simulink model "irep_force_control_m15"  (R2015a)
settings: Solver=ode3  StartTime=0.0  StopTime=inf  FixedStep=dt  RelTol=1e-3
InitFcn:
  | IREP_DEPENDENCY
  | init_omni
  | init_filters
  | init_invivo
  | init_telemanipulation
  | init_parker_xyz
  | init_magnetic_tracker
  | init_loadcell
  | init_scopes
  | init_homing
  | init_force_control
  | init_xpc_invivo_simu
undefined symbols (not defined in the file): ang_vel_scale, B_simu, beta, camera_home_voltage, counter_offset, dt, dt_trakstar, E_Y, encoder_counts, epsilon_robust_inverse, FS_LUT_TAU, FS_LUT_WE, gear_ratio, HomingFineEps, HomingRoughEps, HomingRoughVelocity, I1_primary, I1_secondary, I2_primary, I2_secondary, irep_parameters_left, irep_parameters_right, joystick_filter_coeffs, K_d, K_i, K_naive_inv, K_p, k_right, L1l, L1r, L2l, L2r, L_zeus, left_arm_home_voltage, left_x0_parallelogram, LeftArmHomingDirectionVector, LeftArmHomingIntGain, lin_vel_scale, LOADCELL_BIAS, LOADCELL_GAIN, max_conf_space_speed, N_joystick, N_pots, N_trakstar, OmegaMax, OmegaMin, orientation_epsilon, position_epsilon, pots_filter_coeffs, q_eps_backlash, quadrature_mode, r, right_arm_home_voltage, RightArmHomingDirectionVector, RightArmHomingIntGain, screw_pitch, statics_param, tau_compression_bias, tau_compression_gains, tau_neutral_deadband ... (+16)
libraries: slrtlib x39, simulink x23, xpcobsoletelib x23, xpcconteclib x23, xpcrtudplib x12, xpcmeasurementcomputinglib x6, dspswit3 x2, dspsigops x1
(part 3 of 7)

== system irep_force_control_m15/In-Vivo System/CONTEC CARDS/Level 3 ==
  note: Contec
      | CNT32-8M (PCI)
      | Inc. Encoder
      | Slot: [2, 11]
      | channel [1,4,5,6,7]
  Mux : Mux  Inputs=5
  camera: open joint : xpcconteclib/Incremental Encoder/CNT32-8M(PCI)   Channel=5  OperationMode=2-phase Input Synchronous Clear Multiply by 4  DigitalFilter=No filtering  PulseInput=TTL level input  Direction=Up in the clockwise direction/Down in the counterclockwise direction  InitialValue=counter_offset_init  LoadInitialValue=on  SampleTime=dt  PciSlot=[2,11]  StartMethod=Model Start  StopMethod=Model Terminate  ZeroClearRising=off  ZeroClearFalling=off  ZeroClearMatch0=off  ZeroClearMatch1=off  PresetRising=off  PresetFalling=off  PresetMatch0=off  PresetMatch1=off  PresetValue=0  Match0Value=0  Match1Value=0  OutputSignalMatch0=off  OutputSignalMatch1=off  OutputSignalAbnormal=off  OutputSignalDigitalFilter=off  OutputSignalAlarm=off  OneShotDuration=10 microseconds  IndexEnable=Disable  IndexLogic=Positive (Active High)  EnableDigitalInput=off  EnableDigitalOutput=off  DigitalOutputInitialValue=None  DigitalOutputFinalValue=None
  camera: open joint1 : xpcconteclib/Incremental Encoder/CNT32-8M(PCI)   Channel=6  OperationMode=2-phase Input Synchronous Clear Multiply by 4  DigitalFilter=No filtering  PulseInput=TTL level input  Direction=Up in the clockwise direction/Down in the counterclockwise direction  InitialValue=counter_offset_init  LoadInitialValue=on  SampleTime=dt  PciSlot=[2,11]  StartMethod=Model Start  StopMethod=Model Terminate  ZeroClearRising=off  ZeroClearFalling=off  ZeroClearMatch0=off  ZeroClearMatch1=off  PresetRising=off  PresetFalling=off  PresetMatch0=off  PresetMatch1=off  PresetValue=0  Match0Value=0  Match1Value=0  OutputSignalMatch0=off  OutputSignalMatch1=off  OutputSignalAbnormal=off  OutputSignalDigitalFilter=off  OutputSignalAlarm=off  OneShotDuration=10 microseconds  IndexEnable=Disable  IndexLogic=Positive (Active High)  EnableDigitalInput=off  EnableDigitalOutput=off  DigitalOutputInitialValue=None  DigitalOutputFinalValue=None
  camera: open joint2 : xpcconteclib/Incremental Encoder/CNT32-8M(PCI)   Channel=7  OperationMode=2-phase Input Synchronous Clear Multiply by 4  DigitalFilter=No filtering  PulseInput=TTL level input  Direction=Up in the clockwise direction/Down in the counterclockwise direction  InitialValue=counter_offset_init  LoadInitialValue=on  SampleTime=dt  PciSlot=[2,11]  StartMethod=Model Start  StopMethod=Model Terminate  ZeroClearRising=off  ZeroClearFalling=off  ZeroClearMatch0=off  ZeroClearMatch1=off  PresetRising=off  PresetFalling=off  PresetMatch0=off  PresetMatch1=off  PresetValue=0  Match0Value=0  Match1Value=0  OutputSignalMatch0=off  OutputSignalMatch1=off  OutputSignalAbnormal=off  OutputSignalDigitalFilter=off  OutputSignalAlarm=off  OneShotDuration=10 microseconds  IndexEnable=Disable  IndexLogic=Positive (Active High)  EnableDigitalInput=off  EnableDigitalOutput=off  DigitalOutputInitialValue=None  DigitalOutputFinalValue=None
  left arm: insertion : xpcconteclib/Incremental Encoder/CNT32-8M(PCI)   Channel=4  OperationMode=2-phase Input Synchronous Clear Multiply by 4  DigitalFilter=No filtering  PulseInput=TTL level input  Direction=Up in the clockwise direction/Down in the counterclockwise direction  InitialValue=counter_offset_init  LoadInitialValue=on  SampleTime=dt  PciSlot=[2,11]  StartMethod=Model Start  StopMethod=Model Terminate  ZeroClearRising=off  ZeroClearFalling=off  ZeroClearMatch0=off  ZeroClearMatch1=off  PresetRising=off  PresetFalling=off  PresetMatch0=off  PresetMatch1=off  PresetValue=0  Match0Value=0  Match1Value=0  OutputSignalMatch0=off  OutputSignalMatch1=off  OutputSignalAbnormal=off  OutputSignalDigitalFilter=off  OutputSignalAlarm=off  OneShotDuration=10 microseconds  IndexEnable=Disable  IndexLogic=Positive (Active High)  EnableDigitalInput=off  EnableDigitalOutput=off  DigitalOutputInitialValue=None  DigitalOutputFinalValue=None
  right arm: insertion : xpcconteclib/Incremental Encoder/CNT32-8M(PCI)   Channel=1  OperationMode=2-phase Input Synchronous Clear Multiply by 4  DigitalFilter=No filtering  PulseInput=TTL level input  Direction=Up in the clockwise direction/Down in the counterclockwise direction  InitialValue=counter_offset_init  LoadInitialValue=on  SampleTime=dt  PciSlot=[2,11]  StartMethod=Model Start  StopMethod=Model Terminate  ZeroClearRising=off  ZeroClearFalling=off  ZeroClearMatch0=off  ZeroClearMatch1=off  PresetRising=on  PresetFalling=off  PresetMatch0=off  PresetMatch1=off  PresetValue=0  Match0Value=0  Match1Value=0  OutputSignalMatch0=off  OutputSignalMatch1=off  OutputSignalAbnormal=off  OutputSignalDigitalFilter=off  OutputSignalAlarm=off  OneShotDuration=10 microseconds  IndexEnable=Disable  IndexLogic=Positive (Active High)  EnableDigitalInput=off  EnableDigitalOutput=off  DigitalOutputInitialValue=None  DigitalOutputFinalValue=None
  Out1 : Outport
  wires:
  Mux/1 -> Out1/1
  right arm: insertion/1 -> Mux/1
  camera: open joint2/1 -> Mux/5
  camera: open joint/1 -> Mux/3
  left arm: insertion/1 -> Mux/2
  camera: open joint1/1 -> Mux/4

== system irep_force_control_m15/In-Vivo System/CONTEC CARDS/RZ ==
  note: Contec
      | CNT32-8M (PCI)
      | Inc. Encoder
      | Slot: [2, 14]
      | channel [1,2]
  CNT32-8M(PCI) Ch1 : xpcconteclib/Incremental Encoder/CNT32-8M(PCI)   Channel=1  OperationMode=2-phase Input Synchronous Clear Multiply by 4  DigitalFilter=No filtering  PulseInput=Differential line receiver input  Direction=Up in the clockwise direction/Down in the counterclockwise direction  InitialValue=counter_offset  LoadInitialValue=on  SampleTime=dt  PciSlot=[2 14]  StartMethod=Model Start  StopMethod=Model Terminate  ZeroClearRising=off  ZeroClearFalling=off  ZeroClearMatch0=off  ZeroClearMatch1=off  PresetRising=off  PresetFalling=off  PresetMatch0=off  PresetMatch1=off  PresetValue=0  Match0Value=0  Match1Value=0  OutputSignalMatch0=off  OutputSignalMatch1=off  OutputSignalAbnormal=off  OutputSignalDigitalFilter=off  OutputSignalAlarm=off  OneShotDuration=10 microseconds  IndexEnable=Disable  IndexLogic=Positive (Active High)  EnableDigitalInput=off  EnableDigitalOutput=off  DigitalOutputInitialValue=None  DigitalOutputFinalValue=None
  CNT32-8M(PCI) Ch2 : xpcconteclib/Incremental Encoder/CNT32-8M(PCI)   Channel=2  OperationMode=2-phase Input Synchronous Clear Multiply by 4  DigitalFilter=No filtering  PulseInput=Differential line receiver input  Direction=Up in the clockwise direction/Down in the counterclockwise direction  InitialValue=counter_offset  LoadInitialValue=on  SampleTime=dt  PciSlot=[2 14]  StartMethod=Model Start  StopMethod=Model Terminate  ZeroClearRising=off  ZeroClearFalling=off  ZeroClearMatch0=off  ZeroClearMatch1=off  PresetRising=off  PresetFalling=off  PresetMatch0=off  PresetMatch1=off  PresetValue=0  Match0Value=0  Match1Value=0  OutputSignalMatch0=off  OutputSignalMatch1=off  OutputSignalAbnormal=off  OutputSignalDigitalFilter=off  OutputSignalAlarm=off  OneShotDuration=10 microseconds  IndexEnable=Disable  IndexLogic=Positive (Active High)  EnableDigitalInput=off  EnableDigitalOutput=off  DigitalOutputInitialValue=None  DigitalOutputFinalValue=None
  Mux : Mux  Inputs=2
  Out1 : Outport
  wires:
  Mux/1 -> Out1/1
  CNT32-8M(PCI) Ch1/1 -> Mux/1
  CNT32-8M(PCI) Ch2/1 -> Mux/2

== system irep_force_control_m15/In-Vivo System/Count to mm/Bus Creator ==
  In1 : Inport
  Bus Creator : BusCreator  Inputs=23
  Demux : Demux  Outputs=23
  Out1 : Outport
  wires:
  Demux/1 -> Bus Creator/1  "Righ arm - Proximal segment - bending in Y"
  Demux/2 -> Bus Creator/2  "Right arm - Gripper Joint"
  Demux/3 -> Bus Creator/3  "Right arm - Proximal segment - bending in X"
  Demux/4 -> Bus Creator/4  "Right arm - distal segment - bending in X"
  Demux/5 -> Bus Creator/5  "Right arm - wrist"
  Demux/6 -> Bus Creator/6  "Right arm - distal segment - bending in Y"
  Demux/7 -> Bus Creator/7  "Right arm - parallelogram deployment joint"
  Demux/8 -> Bus Creator/8  "Right arm - parallelogram insert joint"
  Demux/9 -> Bus Creator/9  "Left arm - proximal segment - bending in Y"
  Demux/10 -> Bus Creator/10  "Left arm - gripper joint"
  Demux/11 -> Bus Creator/11  "Left arm - proximal segment - bending in X"
  Demux/12 -> Bus Creator/12  "Left arm - distal segment - bending in x"
  Demux/13 -> Bus Creator/13  "Left arm - wrist"
  Demux/14 -> Bus Creator/14  "Left arm - distal segment - bending in y"
  Demux/15 -> Bus Creator/15  "Left arm - parallelogram deployment joint"
  Demux/16 -> Bus Creator/16  "Left arm - parallelogram insert joint"
  Demux/17 -> Bus Creator/17  "Right arm - overall translational movement"
  Demux/18 -> Bus Creator/18  "Left arm - overall translational movement"
  Demux/19 -> Bus Creator/19  "Camera shell open"
  Demux/20 -> Bus Creator/20  "Camera Pan"
  Demux/21 -> Bus Creator/21  "Camera Tilt"
  Bus Creator/1 -> Out1/1
  In1/1 -> Demux/1
  Demux/22 -> Bus Creator/22  "Parker insertion stage"
  Demux/23 -> Bus Creator/23  "Parker rotary stage"

== system irep_force_control_m15/In-Vivo System/D//A/Bus Selector 1 ==
  In1 : Inport
  Bus Selector : BusSelector  OutputSignals=Right arm - Proximal Segment Y,Right arm - Gripper Joint,Right arm - Proximal Segment X,Right arm - Distal Segment X,Right arm - Wrist Joint,Right arm - Distal Segment Y,Right arm - Parallelogram Deploy,Right arm - Parallelogram Insert
  Gain{,1..3} (4 alike) : Gain  Gain=-1
  Mux : Mux  Inputs=8
  Out1 : Outport
  wires:
  Bus Selector/1 -> Mux/1  "<Right arm - Proximal Segment Y>"
  Bus Selector/2 -> Mux/2  "<Right arm - Gripper Joint>"
  Bus Selector/3 -> Gain/1  "<Right arm - Proximal Segment X>"
  Bus Selector/4 -> Gain1/1  "<Right arm - Distal Segment X>"
  Bus Selector/5 -> Mux/5  "<Right arm - Wrist Joint>"
  Bus Selector/6 -> Mux/6  "<Right arm - Distal Segment Y>"
  Bus Selector/7 -> Gain2/1  "<Right arm - Parallelogram Deploy>"
  Bus Selector/8 -> Gain3/1  "<Right arm - Parallelogram Insert>"
  In1/1 -> Bus Selector/1
  Mux/1 -> Out1/1
  Gain/1 -> Mux/3
  Gain1/1 -> Mux/4
  Gain2/1 -> Mux/7
  Gain3/1 -> Mux/8

== system irep_force_control_m15/In-Vivo System/D//A/Bus Selector 2 ==
  In1 : Inport
  Bus Selector : BusSelector  OutputSignals=Left arm - Proximal Segment Y,Left arm - Gripper Joint,Left arm - Proximal Segment X,Left arm - Distal Segment X,Left arm - Wrist Joint,Left arm - Distal Segment Y,Left arm - Parallelogram Deploy,Left arm - Parallelogram Insert
  Gain{1..4} (4 alike) : Gain  Gain=-1
  Mux : Mux  Inputs=8
  Out1 : Outport
  wires:
  Bus Selector/1 -> Gain1/1  "<Left arm - Proximal Segment Y>"
  Bus Selector/2 -> Mux/2  "<Left arm - Gripper Joint>"
  Bus Selector/4 -> Mux/4  "<Left arm - Distal Segment X>"
  Bus Selector/5 -> Mux/5  "<Left arm - Wrist Joint>"
  Bus Selector/6 -> Gain2/1  "<Left arm - Distal Segment Y>"
  Bus Selector/7 -> Gain3/1  "<Left arm - Parallelogram Deploy>"
  Bus Selector/8 -> Gain4/1  "<Left arm - Parallelogram Insert>"
  In1/1 -> Bus Selector/1
  Mux/1 -> Out1/1
  Bus Selector/3 -> Mux/3  "<Left arm - Proximal Segment X>"
  Gain1/1 -> Mux/1
  Gain2/1 -> Mux/6
  Gain3/1 -> Mux/7
  Gain4/1 -> Mux/8

== system irep_force_control_m15/In-Vivo System/D//A/Bus Selector 3 ==
  In1 : Inport
  Bus Selector : BusSelector  OutputSignals=Righ arm - Overall Translational Movement,Left arm - Overall Translational Movement,Camera shell open,Camera Pan,Camera Tilt
  Mux : Mux  Inputs=5
  Out1 : Outport
  wires:
  Mux/1 -> Out1/1
  In1/1 -> Bus Selector/1
  Bus Selector/1 -> Mux/1  "<Righ arm - Overall Translational Movement>"
  Bus Selector/2 -> Mux/2  "<Left arm - Overall Translational Movement>"
  Bus Selector/3 -> Mux/3  "<Camera shell open>"
  Bus Selector/4 -> Mux/4  "<Camera Pan>"
  Bus Selector/5 -> Mux/5  "<Camera Tilt>"

== system irep_force_control_m15/In-Vivo System/D//A/Level 1 ==
  note: Measurement Computing
      | PCI-DDA08/12 Analog Output
      | slot: [2, 7]
  In1 : Inport
  Demux1 : Demux  Outputs=8
  Level 1 : xpcmeasurementcomputinglib/D//A/PCI-DDA08 12   channel=[1,2,3,4,5,6,7,8]  range=[-10,-10,-10,-10,-10,-10,-10,-10]  reset=[1,1,1,1,1,1,1,1]  initValue=[0,0,0,0,0,0,0,0]  sampletime=dt  pci_dev=[2, 7]
  wires:
  In1/1 -> Demux1/1
  Demux1/1 -> Level 1/1
  Demux1/2 -> Level 1/2
  Demux1/3 -> Level 1/3
  Demux1/4 -> Level 1/4
  Demux1/5 -> Level 1/5
  Demux1/6 -> Level 1/6
  Demux1/7 -> Level 1/7
  Demux1/8 -> Level 1/8

== system irep_force_control_m15/In-Vivo System/D//A/Level 2 ==
  note: Measurement Computing
      | PCI-DDA08/12 Analog Output
      | Slot: [2, 10]
  In1 : Inport
  Demux2 : Demux  Outputs=8
  Level 2 : xpcmeasurementcomputinglib/D//A/PCI-DDA08 12   channel=[1,2,3,4,5,6,7,8]  range=[-10,-10,-10,-10,-10,-10,-10,-10]  reset=[1,1,1,1,1,1,1,1]  initValue=[0,0,0,0,0,0,0,0]  sampletime=dt  pci_dev=[2, 10]
  wires:
  In1/1 -> Demux2/1
  Demux2/1 -> Level 2/1
  Demux2/2 -> Level 2/2
  Demux2/3 -> Level 2/3
  Demux2/4 -> Level 2/4
  Demux2/5 -> Level 2/5
  Demux2/6 -> Level 2/6
  Demux2/7 -> Level 2/7
  Demux2/8 -> Level 2/8

== system irep_force_control_m15/In-Vivo System/D//A/Level 3 ==
  note: Measurement Computing
      | PCI-DDA08/12
      | Analog Ouput
      | Slot: [2, 13]
      | Channels [1,4,5,6,7]
  In1 : Inport
  Demux1 : Demux  Outputs=5
  Level 3 : xpcmeasurementcomputinglib/D//A/PCI-DDA08 12   channel=[1,2,3,4,5,6,7]  range=[-10,-10,-10,-10,-10,-10,-10]  reset=[1,1,1,1,1,1,1]  initValue=[0,0,0,0,0,0,0]  sampletime=dt  pci_dev=[2, 13]
  wires:
  In1/1 -> Demux1/1
  Demux1/1 -> Level 3/1
  Demux1/2 -> Level 3/4
  Demux1/3 -> Level 3/5
  Demux1/4 -> Level 3/6
  Demux1/5 -> Level 3/7

== system irep_force_control_m15/In-Vivo System/D//A/Parker Level ==
  note: Measurement Computing
      | PCI-DAS1602/12
      | Analog Output
      | Slot: [1, 14]
  In1 : Inport
  Bus Selector : BusSelector  OutputSignals=Parker insertion stage,Parker rotary stage
  Gain : Gain  Gain=-1
  Gain1 : Gain  Gain=-1
  "PCI-DAS1602 12 " : xpcobsoletelib/Measurement Computing obs/D//A/PCI-DAS1602 12   channel=[1 2]  range=[-10 -10]  reset=[1 1]  initValue=[0 0]  sampletime=dt  pci_dev=[1 14]
  wires:
  Bus Selector/2 -> Gain/1  "<Parker rotary stage>"
  Bus Selector/1 -> Gain1/1  "<Parker insertion stage>"
  In1/1 -> Bus Selector/1
  Gain1/1 -> "PCI-DAS1602 12 "/1
  Gain/1 -> "PCI-DAS1602 12 "/2

== system irep_force_control_m15/In-Vivo System/Loadcells/Loadcell Backbone Mapping ==
  note: This direction gain is needed for the following reason:
      | The load cell reading "+" meaning tension, i.e. pushing on the backbone.
      | Pushing in the statics formulation use "-".
      | So the loadcell sign is opposite to the statics formulation
  note: This mapping is documented on the wiki
      | http://arma.vuse.vanderbilt.edu/mediawiki/index.php/Force_Sensing,_In-Vivo_Project#Loadcell__Backbone_Mapping
  loadcell reading : Inport
  Demux : Demux  Outputs=8
  Mux : Mux  Inputs=8
  direction : Gain  Gain=-1
  tau backbones : Outport
  wires:
  loadcell reading/1 -> Demux/1
  Demux/1 -> [LC1]  "LC1"
  Demux/2 -> [LC2]  "LC2"
  Demux/3 -> [LC3]  "LC3"
  Demux/4 -> [LC4]  "LC4"
  Demux/5 -> [LC5]  "LC5"
  Demux/6 -> [LC6]  "LC6"
  Demux/7 -> [LC7]  "LC7"
  Demux/8 -> [LC8]  "LC8"
  [LC1] -> Mux/1  "Seg1 BB1"
  [LC4] -> Mux/2  "Seg1 BB2"
  [LC2] -> Mux/3  "Seg1 BB3"
  [LC3] -> Mux/4  "Seg1 BB4"
  [LC8] -> Mux/5  "Seg2 BB1"
  [LC5] -> Mux/6  "Seg2 BB2"
  [LC7] -> Mux/7  "Seg2 BB3"
  [LC6] -> Mux/8  "Seg2 BB4"
  Mux/1 -> direction/1
  direction/1 -> tau backbones/1

== system irep_force_control_m15/In-Vivo System/Magnetic Tracker 125 Hz/process trak1 ==
  raw : Inport
  Filter1 : Subsystem
  Gain : Gain  Gain=[25.4 25.4 25.4 1 1 1]  SampleTime=dt_trakstar
  tracker inversion : Gain  Gain=[-1 -1 -1 -1 -1 -1]  SampleTime=dt_trakstar
  trakstar_to_pose : MATLAB Function  TreatAsAtomicUnit=on
  sensor_pose : Outport
  wires:
  Gain/1 -> Filter1/1(in)
  Filter1/1(out) -> trakstar_to_pose/1(u)
  raw/1 -> Gain/1
  trakstar_to_pose/1(sensor) -> tracker inversion/1
  tracker inversion/1 -> sensor_pose/1

== system irep_force_control_m15/In-Vivo System/Magnetic Tracker 125 Hz/process trak2 ==
  raw : Inport
  Filter1 : Subsystem
  Gain : Gain  Gain=[25.4 25.4 25.4 1 1 1]  SampleTime=dt_trakstar
  trakstar_to_pose : MATLAB Function  TreatAsAtomicUnit=on
  sensor_pose : Outport
  wires:
  trakstar_to_pose/1(sensor) -> sensor_pose/1
  raw/1 -> Gain/1
  Filter1/1(out) -> trakstar_to_pose/1(u)
  Gain/1 -> Filter1/1(in)

== system irep_force_control_m15/In-Vivo System/Magnetic Tracker 125 Hz/process trak3 ==
  raw : Inport
  Filter1 : Subsystem
  Gain : Gain  Gain=[25.4 25.4 25.4 1 1 1]  SampleTime=dt_trakstar
  trakstar_to_pose : MATLAB Function  TreatAsAtomicUnit=on
  sensor_pose : Outport
  wires:
  Gain/1 -> Filter1/1(in)
  Filter1/1(out) -> trakstar_to_pose/1(u)
  raw/1 -> Gain/1
  trakstar_to_pose/1(sensor) -> sensor_pose/1

== system irep_force_control_m15/In-Vivo System/Magnetic Tracker 125 Hz/process trak4 ==
  raw : Inport
  Filter1 : Subsystem
  Gain : Gain  Gain=[25.4 25.4 25.4 1 1 1]  SampleTime=dt_trakstar
  trakstar_to_pose : MATLAB Function  TreatAsAtomicUnit=on
  sensor_pose : Outport
  wires:
  trakstar_to_pose/1(sensor) -> sensor_pose/1
  raw/1 -> Gain/1
  Filter1/1(out) -> trakstar_to_pose/1(u)
  Gain/1 -> Filter1/1(in)

== system irep_force_control_m15/In-Vivo System/Potentiometers/Filter ==
  in : Inport
  Discrete FIR Filter : DiscreteFir  CoefSource=Input port  AccumDataTypeStr=Inherit: Same as product output
  Gain : Gain  Gain=1/N_pots
  vel_filter_coeffs : Constant  Value=pots_filter_coeffs
  out : Outport
  wires:
  in/1 -> Discrete FIR Filter/1
  Gain/1 -> out/1
  vel_filter_coeffs/1 -> Discrete FIR Filter/2
  Discrete FIR Filter/1 -> Gain/1

== system irep_force_control_m15/In-Vivo System/Potentiometers/Filter1 ==
  in : Inport
  Discrete FIR Filter : DiscreteFir  CoefSource=Input port  AccumDataTypeStr=Inherit: Same as product output
  Gain : Gain  Gain=1/N_pots
  vel_filter_coeffs : Constant  Value=pots_filter_coeffs
  out : Outport
  wires:
  Discrete FIR Filter/1 -> Gain/1
  vel_filter_coeffs/1 -> Discrete FIR Filter/2
  Gain/1 -> out/1
  in/1 -> Discrete FIR Filter/1

== system irep_force_control_m15/In-Vivo System/Potentiometers/Filter2 ==
  in : Inport
  Discrete FIR Filter : DiscreteFir  CoefSource=Input port  AccumDataTypeStr=Inherit: Same as product output
  Gain : Gain  Gain=1/N_pots
  vel_filter_coeffs : Constant  Value=pots_filter_coeffs
  out : Outport
  wires:
  Discrete FIR Filter/1 -> Gain/1
  vel_filter_coeffs/1 -> Discrete FIR Filter/2
  Gain/1 -> out/1
  in/1 -> Discrete FIR Filter/1

== system irep_force_control_m15/In-Vivo System/Potentiometers/Filter3 ==
  in : Inport
  Discrete FIR Filter : DiscreteFir  CoefSource=Input port  AccumDataTypeStr=Inherit: Same as product output
  Gain : Gain  Gain=1/N_joystick
  vel_filter_coeffs : Constant  Value=joystick_filter_coeffs
  out : Outport
  wires:
  in/1 -> Discrete FIR Filter/1
  Gain/1 -> out/1
  vel_filter_coeffs/1 -> Discrete FIR Filter/2
  Discrete FIR Filter/1 -> Gain/1

== system irep_force_control_m15/In-Vivo System/Potentiometers/Initialize Joystick ==
  In1 : Inport
  Digital Clock : DigitalClock  SampleTime=dt
  Embedded MATLAB Function : MATLAB Function  TreatAsAtomicUnit=on
  Unit Delay : UnitDelay  InitialCondition=zeros(3,1)  SampleTime=dt
  Out1 : Outport
  wires:
  Digital Clock/1 -> Embedded MATLAB Function/2(t)
  Unit Delay/1 -> Embedded MATLAB Function/3(u_prev)
  In1/1 -> Embedded MATLAB Function/1(u_curr)
  Embedded MATLAB Function/1(V) -> Out1/1  "camer"
  Embedded MATLAB Function/2(v_zero) -> Unit Delay/1  "camera joystick"

== system irep_force_control_m15/In-Vivo System/motor simulation/Bus Creator ==
  In1 : Inport
  Bus Creator : BusCreator  Inputs=23
  Demux : Demux  Outputs=23
  Out1 : Outport
  wires:
  Demux/23 -> Bus Creator/23  "Parker rotary stage"
  Demux/22 -> Bus Creator/22  "Parker insertion stage"
  In1/1 -> Demux/1
  Bus Creator/1 -> Out1/1
  Demux/21 -> Bus Creator/21  "Camera Tilt"
  Demux/20 -> Bus Creator/20  "Camera Pan"
  Demux/19 -> Bus Creator/19  "Camera shell open"
  Demux/18 -> Bus Creator/18  "Left arm - overall translational movement"
  Demux/17 -> Bus Creator/17  "Right arm - overall translational movement"
  Demux/16 -> Bus Creator/16  "Left arm - parallelogram insert joint"
  Demux/15 -> Bus Creator/15  "Left arm - parallelogram deployment joint"
  Demux/14 -> Bus Creator/14  "Left arm - distal segment - bending in y"
  Demux/13 -> Bus Creator/13  "Left arm - wrist"
  Demux/12 -> Bus Creator/12  "Left arm - distal segment - bending in x"
  Demux/11 -> Bus Creator/11  "Left arm - proximal segment - bending in X"
  Demux/10 -> Bus Creator/10  "Left arm - gripper joint"
  Demux/9 -> Bus Creator/9  "Left arm - proximal segment - bending in Y"
  Demux/8 -> Bus Creator/8  "Right arm - parallelogram insert joint"
  Demux/7 -> Bus Creator/7  "Right arm - parallelogram deployment joint"
  Demux/6 -> Bus Creator/6  "Right arm - distal segment - bending in Y"
  Demux/5 -> Bus Creator/5  "Right arm - wrist"
  Demux/4 -> Bus Creator/4  "Right arm - distal segment - bending in X"
  Demux/3 -> Bus Creator/3  "Right arm - Proximal segment - bending in X"
  Demux/2 -> Bus Creator/2  "Right arm - Gripper Joint"
  Demux/1 -> Bus Creator/1  "Righ arm - Proximal segment - bending in Y"

== system irep_force_control_m15/In-Vivo System/motor simulation/motor simu ==
  u : Inport
  Discrete-Time Integrator : DiscreteIntegrator  InitialCondition=zeros(23,1)  SampleTime=dt
  Discrete-Time Integrator1 : DiscreteIntegrator  InitialCondition=zeros(23,1)  SampleTime=dt
  Gain : Gain  Gain=1./B_simu
  q cur : Outport
  wires:
  Gain/1 -> Discrete-Time Integrator/1
  u/1 -> Gain/1
  Discrete-Time Integrator1/1 -> q cur/1
  Discrete-Time Integrator/1 -> Discrete-Time Integrator1/1

== system irep_force_control_m15/In-Vivo System/motor simulation/q_des to q_cur mapping ==
  q cur in : Inport
  Bus Creator1 : BusCreator  Inputs=23
  Bus Selector : BusSelector  OutputSignals=Right arm - Proximal Segment Y,Right arm - Gripper Joint,Right arm - Proximal Segment X,Right arm - Distal Segment X,Right arm - Wrist Joint,Right arm - Distal Segment Y,Right arm - Parallelogram Deploy,Right arm - Parallelogram Insert,Left arm - Proximal Segment Y,Left arm - Gripper Joint,Left arm - Proximal Segment X,Left arm - Distal Segment X,Left arm - Wrist Joint,Left arm - Distal Segment Y,Left arm - Parallelogram Deploy,Left arm - Parallelogram Insert,Righ arm - Overall Translational Movement,Left arm - Overall Translational Movement,Camera shell open,Camera Pan,Camera Tilt,Parker insertion stage,Parker rotary stage
  Demux : Demux  Outputs=23
  Mux : Mux  Inputs=23
  q cur out : Outport
  wires:
  Demux/1 -> Bus Creator1/1  "Righ arm - Overall Translational Movement"
  Demux/2 -> Bus Creator1/2  "Right arm - Parallelogram Insert"
  Demux/3 -> Bus Creator1/3  "Right arm - Parallelogram Deploy"
  Demux/4 -> Bus Creator1/4  "Right arm - Proximal Segment X"
  Demux/5 -> Bus Creator1/5  "Right arm - Proximal Segment Y"
  Demux/6 -> Bus Creator1/6  "Right arm - Distal Segment X"
  Demux/7 -> Bus Creator1/7  "Right arm - Distal Segment Y"
  Demux/8 -> Bus Creator1/8  "Right arm - Wrist Joint"
  Demux/9 -> Bus Creator1/9  "Right arm - Gripper Joint"
  Demux/10 -> Bus Creator1/10  "Left arm - Overall Translational Movement"
  Demux/11 -> Bus Creator1/11  "Left arm - Parallelogram Insert"
  Demux/12 -> Bus Creator1/12  "Left arm - Parallelogram Deploy"
  Demux/13 -> Bus Creator1/13  "Left arm - Proximal Segment X"
  Demux/14 -> Bus Creator1/14  "Left arm - Proximal Segment Y"
  Demux/15 -> Bus Creator1/15  "Left arm - Distal Segment X"
  Demux/16 -> Bus Creator1/16  "Left arm - Distal Segment Y"
  Demux/17 -> Bus Creator1/17  "Left arm - Wrist Joint"
  Demux/18 -> Bus Creator1/18  "Left arm - Gripper Joint"
  Demux/19 -> Bus Creator1/19  "Camera shell open"
  Demux/20 -> Bus Creator1/20  "Camera Pan"
  Demux/21 -> Bus Creator1/21  "Camera Tilt"
  Demux/22 -> Bus Creator1/22  "Parker insertion stage"
  Demux/23 -> Bus Creator1/23  "Parker rotary stage"
  Bus Creator1/1 -> Bus Selector/1
  Bus Selector/1 -> Mux/1  "<Right arm - Proximal Segment Y>"
  Bus Selector/2 -> Mux/2  "<Right arm - Gripper Joint>"
  Bus Selector/3 -> Mux/3  "<Right arm - Proximal Segment X>"
  Bus Selector/4 -> Mux/4  "<Right arm - Distal Segment X>"
  Bus Selector/5 -> Mux/5  "<Right arm - Wrist Joint>"
  Bus Selector/6 -> Mux/6  "<Right arm - Distal Segment Y>"
  Bus Selector/7 -> Mux/7  "<Right arm - Parallelogram Deploy>"
  Bus Selector/8 -> Mux/8  "<Right arm - Parallelogram Insert>"
  Bus Selector/9 -> Mux/9  "<Left arm - Proximal Segment Y>"
  Bus Selector/10 -> Mux/10  "<Left arm - Gripper Joint>"
  Bus Selector/11 -> Mux/11  "<Left arm - Proximal Segment X>"
  Bus Selector/12 -> Mux/12  "<Left arm - Distal Segment X>"
  Bus Selector/13 -> Mux/13  "<Left arm - Wrist Joint>"
  Bus Selector/14 -> Mux/14  "<Left arm - Distal Segment Y>"
  Bus Selector/15 -> Mux/15  "<Left arm - Parallelogram Deploy>"
  Bus Selector/16 -> Mux/16  "<Left arm - Parallelogram Insert>"
  Bus Selector/17 -> Mux/17  "<Righ arm - Overall Translational Movement>"
  Bus Selector/18 -> Mux/18  "<Left arm - Overall Translational Movement>"
  Bus Selector/19 -> Mux/19  "<Camera shell open>"
  Bus Selector/20 -> Mux/20  "<Camera Pan>"
  Bus Selector/21 -> Mux/21  "<Camera Tilt>"
  Bus Selector/22 -> Mux/22  "<Parker insertion stage>"
  Bus Selector/23 -> Mux/23  "<Parker rotary stage>"
  q cur in/1 -> Demux/1
  Mux/1 -> q cur out/1

== system irep_force_control_m15/In-Vivo System/motor simulation/u mapping ==
  u in : Inport
  Bus Selector : BusSelector  OutputSignals=Righ arm - Overall Translational Movement,Right arm - Parallelogram Insert,Right arm - Parallelogram Deploy,Right arm - Proximal Segment X,Right arm - Proximal Segment Y,Right arm - Distal Segment X,Right arm - Distal Segment Y,Right arm - Wrist Joint,Right arm - Gripper Joint,Left arm - Overall Translational Movement,Left arm - Parallelogram Insert,Left arm - Parallelogram Deploy,Left arm - Proximal Segment X,Left arm - Proximal Segment Y,Left arm - Distal Segment X,Left arm - Distal Segment Y,Left arm - Wrist Joint,Left arm - Gripper Joint,Camera shell open,Camera Pan,Camera Tilt,Parker insertion stage,Parker rotary stage
  Mux : Mux  Inputs=23
  u out : Outport
  wires:
  Bus Selector/1 -> Mux/1  "<Righ arm - Overall Translational Movement>"
  Bus Selector/2 -> Mux/2  "<Right arm - Parallelogram Insert>"
  Bus Selector/3 -> Mux/3  "<Right arm - Parallelogram Deploy>"
  Bus Selector/4 -> Mux/4  "<Right arm - Proximal Segment X>"
  Bus Selector/5 -> Mux/5  "<Right arm - Proximal Segment Y>"
  Bus Selector/6 -> Mux/6  "<Right arm - Distal Segment X>"
  Bus Selector/7 -> Mux/7  "<Right arm - Distal Segment Y>"
  Bus Selector/8 -> Mux/8  "<Right arm - Wrist Joint>"
  Bus Selector/9 -> Mux/9  "<Right arm - Gripper Joint>"
  Bus Selector/10 -> Mux/10  "<Left arm - Overall Translational Movement>"
  Bus Selector/11 -> Mux/11  "<Left arm - Parallelogram Insert>"
  Bus Selector/12 -> Mux/12  "<Left arm - Parallelogram Deploy>"
  Bus Selector/13 -> Mux/13  "<Left arm - Proximal Segment X>"
  Bus Selector/14 -> Mux/14  "<Left arm - Proximal Segment Y>"
  Bus Selector/15 -> Mux/15  "<Left arm - Distal Segment X>"
  Bus Selector/16 -> Mux/16  "<Left arm - Distal Segment Y>"
  Bus Selector/17 -> Mux/17  "<Left arm - Wrist Joint>"
  Bus Selector/18 -> Mux/18  "<Left arm - Gripper Joint>"
  Bus Selector/19 -> Mux/19  "<Camera shell open>"
  Bus Selector/20 -> Mux/20  "<Camera Pan>"
  Bus Selector/21 -> Mux/21  "<Camera Tilt>"
  Bus Selector/22 -> Mux/22  "<Parker insertion stage>"
  Bus Selector/23 -> Mux/23  "<Parker rotary stage>"
  u in/1 -> Bus Selector/1
  Mux/1 -> u out/1

== system irep_force_control_m15/Joint Level PID Control in mm/Bus selector/Camera selector ==
  In1 : Inport
  Bus Selector : BusSelector  OutputSignals=q.Camera shell open,q.Camera Pan,q.Camera Tilt
  Mux : Mux  Inputs=3
  Out1 : Outport
  wires:
  Mux/1 -> Out1/1
  In1/1 -> Bus Selector/1
  Bus Selector/3 -> Mux/3  "<Camera Tilt>"
  Bus Selector/2 -> Mux/2  "<Camera Pan>"
  Bus Selector/1 -> Mux/1  "<Camera shell open>"

== system irep_force_control_m15/Joint Level PID Control in mm/Bus selector/Left arm selector ==
  In1 : Inport
  Bus Selector : BusSelector  OutputSignals=q.Left arm - overall translational movement,q.Left arm - parallelogram insert joint,q.Left arm - parallelogram deployment joint,q.Left arm - proximal segment - bending in X,q.Left arm - proximal segment - bending in Y,q.Left arm - distal segment - bending in x,q.Left arm - distal segment - bending in y,q.Left arm - wrist,q.Left arm - gripper joint
  Mux : Mux  Inputs=9
  Out1 : Outport
  wires:
  In1/1 -> Bus Selector/1
  Mux/1 -> Out1/1
  Bus Selector/1 -> Mux/1  "<Left arm - overall translational movement>"
  Bus Selector/2 -> Mux/2  "<Left arm - parallelogram insert joint>"
  Bus Selector/3 -> Mux/3  "<Left arm - parallelogram deployment joint>"
  Bus Selector/4 -> Mux/4  "<Left arm - proximal segment - bending in X>"
  Bus Selector/5 -> Mux/5  "<Left arm - proximal segment - bending in Y>"
  Bus Selector/8 -> Mux/8  "<Left arm - wrist>"
  Bus Selector/9 -> Mux/9  "<Left arm - gripper joint>"
  Bus Selector/6 -> Mux/6  "<Left arm - distal segment - bending in x>"
  Bus Selector/7 -> Mux/7  "<Left arm - distal segment - bending in y>"

== system irep_force_control_m15/Joint Level PID Control in mm/Bus selector/RZ ==
  In1 : Inport
  Bus Selector : BusSelector  OutputSignals=q.Parker insertion stage,q.Parker rotary stage
  Mux : Mux  Inputs=2
  Out1 : Outport
  wires:
  Mux/1 -> Out1/1
  In1/1 -> Bus Selector/1
  Bus Selector/2 -> Mux/2  "<Parker rotary stage>"
  Bus Selector/1 -> Mux/1  "<Parker insertion stage>"

== system irep_force_control_m15/Joint Level PID Control in mm/Bus selector/Right arm selector ==
  In1 : Inport
  Bus Selector : BusSelector  OutputSignals=q.Right arm - overall translational movement,q.Right arm - parallelogram insert joint,q.Right arm - parallelogram deployment joint,q.Right arm - Proximal segment - bending in X,q.Righ arm - Proximal segment - bending in Y,q.Right arm - distal segment - bending in X,q.Right arm - distal segment - bending in Y,q.Right arm - wrist,q.Right arm - Gripper Joint
  Mux : Mux  Inputs=9
  Out1 : Outport
  wires:
  In1/1 -> Bus Selector/1
  Mux/1 -> Out1/1
  Bus Selector/1 -> Mux/1  "<Right arm - overall translational movement>"
  Bus Selector/2 -> Mux/2  "<Right arm - parallelogram insert joint>"
  Bus Selector/3 -> Mux/3  "<Right arm - parallelogram deployment joint>"
  Bus Selector/4 -> Mux/4  "<Right arm - Proximal segment - bending in X>"
  Bus Selector/5 -> Mux/5  "<Righ arm - Proximal segment - bending in Y>"
  Bus Selector/6 -> Mux/6  "<Right arm - distal segment - bending in X>"
  Bus Selector/7 -> Mux/7  "<Right arm - distal segment - bending in Y>"
  Bus Selector/8 -> Mux/8  "<Right arm - wrist>"
  Bus Selector/9 -> Mux/9  "<Right arm - Gripper Joint>"

== system irep_force_control_m15/Scopes/Friction Estimation Data UDP/Right arm joint def ==
  sensors : Inport
  Bus Selector4 : BusSelector  OutputSignals=q.Right arm - overall translational movement,q.Right arm - parallelogram insert joint,q.Right arm - parallelogram deployment joint,q.Right arm - Proximal segment - bending in X,q.Righ arm - Proximal segment - bending in Y,q.Right arm - distal segment - bending in X,q.Right arm - distal segment - bending in Y,q.Right arm - wrist,q.Right arm - Gripper Joint
  Mux1 : Mux  Inputs=9
  right q_cur : Outport
  wires:
  Bus Selector4/1 -> Mux1/1  "<Right arm - overall translational movement>"
  Bus Selector4/2 -> Mux1/2  "<Right arm - parallelogram insert joint>"
  Bus Selector4/3 -> Mux1/3  "<Right arm - parallelogram deployment joint>"
  Bus Selector4/4 -> Mux1/4  "<Right arm - Proximal segment - bending in X>"
  Bus Selector4/5 -> Mux1/5  "<Righ arm - Proximal segment - bending in Y>"
  Bus Selector4/6 -> Mux1/6  "<Right arm - distal segment - bending in X>"
  Bus Selector4/7 -> Mux1/7  "<Right arm - distal segment - bending in Y>"
  Bus Selector4/8 -> Mux1/8  "<Right arm - wrist>"
  Bus Selector4/9 -> Mux1/9  "<Right arm - Gripper Joint>"
  sensors/1 -> Bus Selector4/1
  Mux1/1 -> right q_cur/1

== system irep_force_control_m15/Trajectory Planner/Camera/Homing Procedure ==
  sensors : Inport
  Enable : EnablePort
  Bus Selector : BusSelector  OutputSignals=A/D signals.camera pots
  Discrete-Time Integrator : DiscreteIntegrator  InitialCondition=zeros(3,1)  SampleTime=dt
  Gain : Gain  Gain=[0.1 0.1 0.1]  SampleTime=dt
  Homing Completion : MATLAB Function  TreatAsAtomicUnit=on
  Sum : Sum  Inputs=|+-  SampleTime=dt
  Terminator1 : Terminator
  home voltage : Constant  Value=camera_home_voltage  SampleTime=dt
  q des : Outport
  wires:
  sensors/1 -> Bus Selector/1
  home voltage/1 -> Sum/1
  Bus Selector/1 -> Sum/2  "<camera pots>"
  Sum/1 -> Gain/1, Homing Completion/1(u)
  Gain/1 -> Discrete-Time Integrator/1
  Discrete-Time Integrator/1 -> q des/1
  Homing Completion/1(y) -> Terminator1/1

== system irep_force_control_m15/Trajectory Planner/Camera/Joint Space ==
  Enable : EnablePort
  q des : Constant  Value=zeros(3,1)  SampleTime=dt
  Out1 : Outport
  wires:
  q des/1 -> Out1/1

== system irep_force_control_m15/Trajectory Planner/Camera/Joystick Control for Cam ==
  sensors : Inport
  Enable : EnablePort
  Bus Selector : BusSelector  OutputSignals=A/D signals.camera joystick
  Demux : Demux  Outputs=3
  Discrete-Time Integrator : DiscreteIntegrator  SampleTime=dt  LimitOutput=on  UpperSaturationLimit=[3;3;3]  LowerSaturationLimit=[-3;-3;-3]
  Gain : Gain  Gain=diag([0.3 0.3 0.3])  Multiplication=Matrix(K*u)  SampleTime=dt
  Gain1 : Gain  Gain=-1
  Mux : Mux  Inputs=3
  q des : Outport
  wires:
  sensors/1 -> Bus Selector/1
  Gain/1 -> Discrete-Time Integrator/1
  Discrete-Time Integrator/1 -> q des/1
  Bus Selector/1 -> Demux/1  "<camera joystick>"
  Mux/1 -> Gain/1
  Demux/2 -> Gain1/1
  Demux/1 -> Mux/2
  Demux/3 -> Mux/1
  Gain1/1 -> Mux/3

== system irep_force_control_m15/Trajectory Planner/Camera/Tool Tracking ==
  tool XY : Inport
  Enable : EnablePort
  Constant1 : Constant  Value=0  SampleTime=dt
  Discrete-Time Integrator : DiscreteIntegrator  SampleTime=dt  LimitOutput=on  UpperSaturationLimit=[3;3]  LowerSaturationLimit=[-3;-3]
  Gain : Gain  Gain=[0.01,0.01]  SampleTime=dt
  Mux : Mux  Inputs=2
  q des : Outport
  wires:
  tool XY/1 -> Gain/1
  Mux/1 -> q des/1
  Constant1/1 -> Mux/1
  Gain/1 -> Discrete-Time Integrator/1
  Discrete-Time Integrator/1 -> Mux/2

== system irep_force_control_m15/Trajectory Planner/Left Arm/High Level ==
  Master : Inport
  sensors : Inport  Port=2
  Enable : EnablePort
  Actuation Compensation : Subsystem  TreatAsAtomicUnit=on
  Add : Sum
  Configuration Space : Subsystem  TreatAsAtomicUnit=on
  Enable Compensation : Constant  Value=0  SampleTime=dt
  Enable Configuration Space : Constant  Value=0  SampleTime=dt
  Enable Task Space : Constant  Value=0  SampleTime=dt
  Inverse Istantaneous Kinematics : Subsystem
  Merge : Merge  InitialOutput=zeros(8,1)
  Task Space : Subsystem  TreatAsAtomicUnit=on
  q des : Outport
  conf space : Outport  Port=2
  b0_dot_left : Outport  Port=3
  TASK_EN : Outport  Port=4
  current_pose : Outport  Port=5
  wires:
  Enable Task Space/1 -> TASK_EN/1, Task Space/Enable
  Task Space/1("b1 dot, psi dot") -> Merge/2
  Master/1 -> Task Space/1(Master), Inverse Istantaneous Kinematics/3(Master)
  Inverse Istantaneous Kinematics/2(conf space) -> Actuation Compensation/2(conf space), Task Space/2("b1 curr, psi curr"), conf space/1
  Inverse Istantaneous Kinematics/1(q des) -> Actuation Compensation/1(q des), Add/1
  Add/1 -> q des/1
  Actuation Compensation/1(epsilon) -> Add/2
  Enable Compensation/1 -> Actuation Compensation/Enable
  Enable Configuration Space/1 -> Configuration Space/Enable
  Configuration Space/1("b1 dot, psi dot") -> Merge/1
  sensors/1 -> Inverse Istantaneous Kinematics/2(sensors), Task Space/3(sensors)
  Merge/1 -> Inverse Istantaneous Kinematics/1(In1)
  Inverse Istantaneous Kinematics/3(b0 dot left) -> b0_dot_left/1
  Task Space/2(current_pose) -> current_pose/1

== system irep_force_control_m15/Trajectory Planner/Left Arm/Low Level ==
  sensors : Inport
  Enable : EnablePort
  Bus Selector : BusSelector  OutputSignals=Pots_Connect.L_Pots_Connect
  Enable Home Procedure : Constant  Value=0  SampleTime=dt
  Enable Joint Space : Constant  Value=0  SampleTime=dt
  Home Procedure : Subsystem  TreatAsAtomicUnit=on
  Joint Space : Subsystem  TreatAsAtomicUnit=on
  Merge1 : Merge  InitialOutput=zeros(9,1)
  Not And : MATLAB Function  TreatAsAtomicUnit=on
  q des : Outport
  wires:
  sensors/1 -> Bus Selector/1, Home Procedure/1(sensors)
  Merge1/1 -> q des/1
  Enable Joint Space/1 -> Joint Space/Enable
  Joint Space/1(q des) -> Merge1/2
  Bus Selector/1 -> Not And/1(connected)  "<L_Pots_Connect>"
  Enable Home Procedure/1 -> Not And/2(enable_home)
  Not And/1(enable) -> Home Procedure/Enable
  Home Procedure/1(q des) -> Merge1/1

== system irep_force_control_m15/Trajectory Planner/RZ/Joystick Control for RZ ==
  sensors : Inport
  Enable : EnablePort
  Bus Selector : BusSelector  OutputSignals=A/D signals.camera joystick
  Embedded MATLAB Function : MATLAB Function  TreatAsAtomicUnit=on
  Gain : Gain  Gain=diag(-[2 0 0.005])  Multiplication=Matrix(K*u)  SampleTime=dt
  q des : Outport
  wires:
  sensors/1 -> Bus Selector/1
  Gain/1 -> q des/1
  Embedded MATLAB Function/1(y) -> Gain/1
  Bus Selector/1 -> Embedded MATLAB Function/1(u)  "<camera joystick>"

== system irep_force_control_m15/Trajectory Planner/RZ/Subsystem ==
  In1 : Inport
  Demux : Demux  Outputs=3
  Mux : Mux  Inputs=2
  Terminator : Terminator
  Out1 : Outport
  wires:
  Demux/1 -> Mux/1
  Demux/3 -> Mux/2
  Demux/2 -> Terminator/1
  In1/1 -> Demux/1
  Mux/1 -> Out1/1

== system irep_force_control_m15/Trajectory Planner/Right Arm/High Level ==
  Master : Inport
  sensors : Inport  Port=2
  Enable : EnablePort
  Actuation Compensation : Subsystem  TreatAsAtomicUnit=on
  Add : Sum
  Configuration Space : Subsystem  TreatAsAtomicUnit=on
  Enable Compensation : Constant  Value=0  SampleTime=dt
  Enable Configuration Space : Constant  Value=0  SampleTime=dt
  Enable Task Space : Constant  Value=0  SampleTime=dt
  Inverse Istantaneous Kinematics : Subsystem
  Merge : Merge  InitialOutput=zeros(8,1)
  Right eps : slrtlib/Displays and Logging/Scope   scopeno=32  scopetype=Host  autostart=on  viewmode=Numerical  formatstr=scope_format_right_q_des  grid=on  ylimits=[0,0]  nosamples=10  noprepostsamples=0  interleave=1  triggermode=FreeRun  triggersignal=1  trigsignalfromport=off  triggerlevel=0.0  triggerslope=Either  triggerscope=1  triggersample=0  filename=weights.dat  mode=Lazy  writesize=512  autorestart=off  dynamicfilemode=off  maxwritefilesize=512*1024^2
  Task Space : Subsystem  TreatAsAtomicUnit=on
  delay : Subsystem
  q des : Outport
  conf space : Outport  Port=2  PortDimensions=8
  b0 dot : Outport  Port=3  PortDimensions=1
  TASK_EN : Outport  Port=4
  current_pose : Outport  Port=5
  q dot sgn : Outport  Port=6
  wires:
  Merge/1 -> [psi_dot], Inverse Istantaneous Kinematics/1(PSI dot)
  Enable Task Space/1 -> TASK_EN/1, Task Space/Enable
  Task Space/1("b0 dot, b1 dot, psi dot") -> Merge/2
  Master/1 -> Task Space/1(Master), Inverse Istantaneous Kinematics/3(Master)
  Inverse Istantaneous Kinematics/2(conf space) -> Actuation Compensation/2(conf space), Task Space/2("b1 curr, psi curr"), conf space/1
  Configuration Space/1("b1 dot, psi dot") -> Merge/1
  Inverse Istantaneous Kinematics/1(q des) -> Add/1, delay/1(In1)
  Actuation Compensation/1(epsilon) -> Add/2, Right eps/1
  Enable Compensation/1 -> Actuation Compensation/Enable
  sensors/1 -> Task Space/3(sensors), Inverse Istantaneous Kinematics/2(sensors)
  Inverse Istantaneous Kinematics/3(b0_dot_right) -> b0 dot/1
  Add/1 -> q des/1
  Task Space/2(current_pose) -> current_pose/1
  Enable Configuration Space/1 -> Configuration Space/Enable
  [psi_dot] -> Actuation Compensation/3(psi dot)
  delay/1(Out1) -> Actuation Compensation/1(q des)
  Actuation Compensation/2(q dot sgn) -> q dot sgn/1

== system irep_force_control_m15/Trajectory Planner/Right Arm/Low Level ==
  sensors : Inport
  Enable : EnablePort
  Bus Selector : BusSelector  OutputSignals=Pots_Connect.R_Pots_Connect
  Enable Home Procedure : Constant  Value=0  SampleTime=dt
  Enable Joint Space : Constant  Value=0  SampleTime=dt
  Home Procedure : Subsystem  TreatAsAtomicUnit=on
  Joint Space : Subsystem  TreatAsAtomicUnit=on
  Merge1 : Merge  InitialOutput=zeros(9,1)
  Not And : MATLAB Function  TreatAsAtomicUnit=on
  q des : Outport
  wires:
  sensors/1 -> Home Procedure/1(sensors), Bus Selector/1
  Home Procedure/1(q des) -> Merge1/1
  Enable Joint Space/1 -> Joint Space/Enable
  Joint Space/1(q des) -> Merge1/2
  Merge1/1 -> q des/1
  Bus Selector/1 -> Not And/1(connected)  "<R_Pots_Connect>"
  Not And/1(enable) -> Home Procedure/Enable
  Enable Home Procedure/1 -> Not And/2(enable_home)

== system irep_force_control_m15/Trajectory Planner/UDP_SendTo_MTM/Left_UDP ==
  traj : Inport
  MTM : Inport  Port=2
  Bus Selector : BusSelector  OutputSignals=left arm.PSM_READY,left arm.current_pose,left arm.q des left
  Bus Selector1 : BusSelector  OutputSignals=p in world,R in world
  Bus Selector2 : BusSelector  OutputSignals=MSG_Type,MTM_time
  Constant : Constant  Value=zeros(6,1)
  Demux : Demux  Outputs=21
  Embedded MATLAB Function : MATLAB Function  TreatAsAtomicUnit=on
  Left_Send : xpcrtudplib/Legacy UDP/Send   ipAddress=192.168.1.104  ipPort=10004  localPort=-1  vblLen=off  sampletime=dt_omni
  MSG_Decoding : MATLAB Function  TreatAsAtomicUnit=on
  Mux : Mux  Inputs=6
  Pack : xpcobsoletelib/Utilities/Pack   datatypes={'double' 'double' 'double' 'double' 'double' 'double' 'double' 'double' 'double' 'double' 'double' 'double' 'double' 'double' 'double' 'double' 'double' 'double' 'double' 'double' 'double'}  byteAlign=1
  Rate Transition2 : RateTransition  OutPortSampleTime=dt_omni
  Sum : Sum  Inputs=|++
  mm to m : Gain  Gain=1/1000
  nothing : Constant  Value=0
  pose convert : Subsystem
  pose_curr_scope : Subsystem
  select q9 : Subsystem
  wires:
  pose convert/1(pose_R) -> Bus Selector1/1, pose_curr_scope/1(left)
  Bus Selector/2 -> pose convert/1(pose_q)  "<current_pose>"
  Constant/1 -> Mux/5  "Wrench"
  Demux/21 -> Pack/21
  Demux/20 -> Pack/20
  Demux/19 -> Pack/19
  Demux/18 -> Pack/18
  Demux/17 -> Pack/17
  Demux/16 -> Pack/16
  Demux/15 -> Pack/15
  Demux/14 -> Pack/14
  Demux/13 -> Pack/13
  Demux/12 -> Pack/12
  Demux/11 -> Pack/11
  Demux/10 -> Pack/10
  Demux/9 -> Pack/9
  Demux/8 -> Pack/8
  Demux/7 -> Pack/7
  Demux/6 -> Pack/6
  Demux/5 -> Pack/5
  Demux/4 -> Pack/4
  Demux/3 -> Pack/3
  Demux/2 -> Pack/2
  Demux/1 -> Pack/1
  [time] -> Mux/6
  Sum/1 -> Mux/1
  [EN] -> Sum/2
  Bus Selector/1 -> Sum/1  "<PSM_READY>"
  nothing/1 -> Mux/2
  MSG_Decoding/1(EN) -> [EN]
  Bus Selector2/2 -> [time]  "<MTM_time>"
  Bus Selector2/1 -> MSG_Decoding/1(MSG_Type)  "<MSG_Type>"
  MTM/1 -> Bus Selector2/1
  select q9/1(q9) -> pose_curr_scope/2(q9)
  Bus Selector/3 -> select q9/1(qdes)  "<q des left>"
  mm to m/1 -> Mux/3
  traj/1 -> Bus Selector/1
  Embedded MATLAB Function/1(R_vec) -> Mux/4
  Bus Selector1/1 -> mm to m/1  "<p in world>"
  Rate Transition2/1 -> Demux/1
  Mux/1 -> Rate Transition2/1
  Pack/1 -> Left_Send/1
  Bus Selector1/2 -> Embedded MATLAB Function/1(R)  "<R in world>"

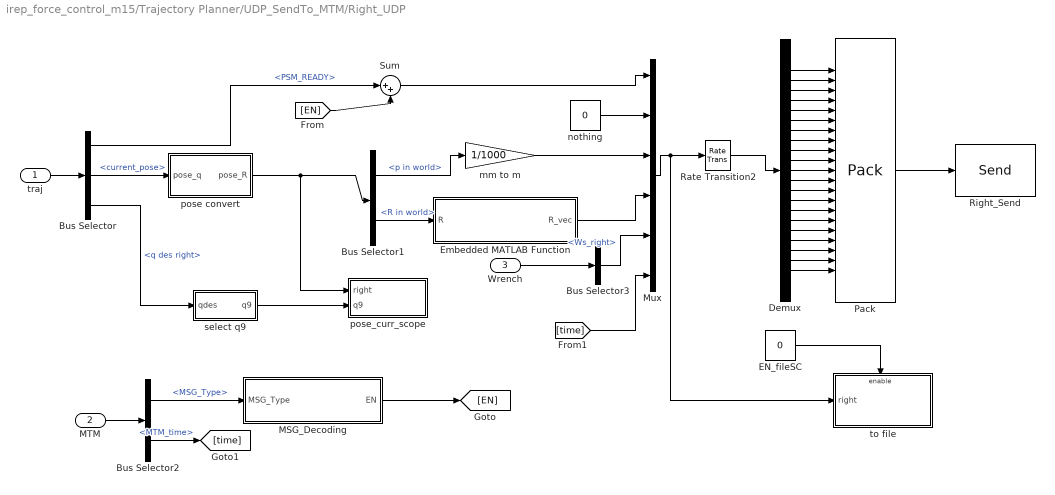
== system irep_force_control_m15/Trajectory Planner/UDP_SendTo_MTM/Right_UDP ==
  traj : Inport
  MTM : Inport  Port=2
  Wrench : Inport  Port=3
  Bus Selector : BusSelector  OutputSignals=right arm.PSM_READY,right arm.current_pose,right arm.q des right
  Bus Selector1 : BusSelector  OutputSignals=p in world,R in world
  Bus Selector2 : BusSelector  OutputSignals=MSG_Type,MTM_time
  Bus Selector3 : BusSelector  OutputSignals=Ws_right
  Demux : Demux  Outputs=21
  EN_fileSC : Constant  Value=0
  Embedded MATLAB Function : MATLAB Function  TreatAsAtomicUnit=on
  MSG_Decoding : MATLAB Function  TreatAsAtomicUnit=on
  Mux : Mux  Inputs=6
  Pack : xpcobsoletelib/Utilities/Pack   datatypes={'double' 'double' 'double' 'double' 'double' 'double' 'double' 'double' 'double' 'double' 'double' 'double' 'double' 'double' 'double' 'double' 'double' 'double' 'double' 'double' 'double'}  byteAlign=1
  Rate Transition2 : RateTransition  OutPortSampleTime=dt_omni
  Right_Send : xpcrtudplib/Legacy UDP/Send   ipAddress=192.168.1.104  ipPort=10005  localPort=-1  vblLen=off  sampletime=dt_omni
  Sum : Sum  Inputs=|++
  mm to m : Gain  Gain=1/1000
  nothing : Constant  Value=0
  pose convert : Subsystem
  pose_curr_scope : Subsystem
  select q9 : Subsystem
  to file : Subsystem
  wires:
  Bus Selector1/2 -> Embedded MATLAB Function/1(R)  "<R in world>"
  Pack/1 -> Right_Send/1
  Mux/1 -> Rate Transition2/1, to file/1(right)
  Rate Transition2/1 -> Demux/1
  Bus Selector1/1 -> mm to m/1  "<p in world>"
  Embedded MATLAB Function/1(R_vec) -> Mux/4
  traj/1 -> Bus Selector/1
  mm to m/1 -> Mux/3
  Bus Selector/3 -> select q9/1(qdes)  "<q des right>"
  select q9/1(q9) -> pose_curr_scope/2(q9)
  MTM/1 -> Bus Selector2/1
  Bus Selector2/1 -> MSG_Decoding/1(MSG_Type)  "<MSG_Type>"
  Bus Selector2/2 -> [time]  "<MTM_time>"
  MSG_Decoding/1(EN) -> [EN]
  EN_fileSC/1 -> to file/Enable
  nothing/1 -> Mux/2
  Bus Selector/1 -> Sum/1  "<PSM_READY>"
  [EN] -> Sum/2
  Sum/1 -> Mux/1
  [time] -> Mux/6
  Demux/1 -> Pack/1
  Demux/2 -> Pack/2
  Demux/3 -> Pack/3
  Demux/4 -> Pack/4
  Demux/5 -> Pack/5
  Demux/6 -> Pack/6
  Demux/7 -> Pack/7
  Demux/8 -> Pack/8
  Demux/9 -> Pack/9
  Demux/10 -> Pack/10
  Demux/11 -> Pack/11
  Demux/12 -> Pack/12
  Demux/13 -> Pack/13
  Demux/14 -> Pack/14
  Demux/15 -> Pack/15
  Demux/16 -> Pack/16
  Demux/17 -> Pack/17
  Demux/18 -> Pack/18
  Demux/19 -> Pack/19
  Demux/20 -> Pack/20
  Demux/21 -> Pack/21
  Wrench/1 -> Bus Selector3/1
  Bus Selector3/1 -> Mux/5  "<Ws_right>"
  Bus Selector/2 -> pose convert/1(pose_q)  "<current_pose>"
  pose convert/1(pose_R) -> Bus Selector1/1, pose_curr_scope/1(right)

== system irep_force_control_m15/Wrench Estimation/Wrench Compensation/wrench sensing compensation LUT ==
  note: 1st Segment tau bias
  note: Wrench est at the tip
  note: Inputs
  q_dot_sign : Inport
  psi : Inport  Port=2
  Enable : EnablePort
  Constant : Constant  Value=zeros(6,1)
  Demux : Demux  Outputs=[4,4]
  Demux1 : Demux  Outputs=[2,2]
  Mux : Mux  Inputs=2
  Terminator : Terminator
  Terminator1 : Terminator
  wrench seg2 bias LUT : Subsystem
  ws_bias : Outport
  wires:
  psi/1 -> Demux1/1
  q_dot_sign/1 -> Demux/1
  Demux1/1 -> [psi1]
  Demux1/2 -> [psi2]
  [psi1] -> Terminator/1
  Demux/1 -> [qdot_sgn1]
  Demux/2 -> [qdot_sgn2]
  [qdot_sgn1] -> Terminator1/1
  [psi2] -> wrench seg2 bias LUT/2(psi seg2)
  [qdot_sgn2] -> wrench seg2 bias LUT/1(q dot seg2)
  Mux/1 -> ws_bias/1
  wrench seg2 bias LUT/1(wrench bias seg2) -> Mux/1
  Constant/1 -> Mux/2

== system irep_force_control_m15/Wrench Estimation/Wrench Est Right Arm/sel param ==
  note: irep_parameters_right = [Y_OFFSET;L1r;L2r;p_gripper];
  In : Inport
  Demux : Demux  Outputs=[1,1,1,3]
  Mux1 : Mux  Inputs=2
  Terminator : Terminator
  Terminator1 : Terminator
  L : Outport
  wires:
  In/1 -> Demux/1
  Mux1/1 -> L/1
  Demux/2 -> Mux1/1  "L1"
  Demux/3 -> Mux1/2  "L2"
  Demux/1 -> Terminator/1  "Y_OFFSET"
  Demux/4 -> Terminator1/1  "p_gripper"

== system irep_force_control_m15/Wrench Estimation/tau sensing compensation/tau sensing compensation LUT ==
  note: 1st Segment tau bias
  note: 2nd Segment tau bias
  note: Inputs
  tau_measured : Inport
  q_dot_sign : Inport  Port=2
  psi : Inport  Port=3
  Enable : EnablePort
  Constant : Constant  Value=zeros(4,1)
  Demux : Demux  Outputs=[4,4]
  Demux1 : Demux  Outputs=[2,2]
  Mux : Mux  Inputs=2
  Sum : Sum  Inputs=|+-
  Terminator : Terminator
  Terminator1 : Terminator
  tau seg2 bias LUT : Subsystem
  tau_comp : Outport
  wires:
  psi/1 -> Demux1/1
  q_dot_sign/1 -> Demux/1
  Demux1/1 -> [psi1]
  Demux1/2 -> [psi2]
  [psi1] -> Terminator/1
  Demux/1 -> [qdot_sgn1]
  Demux/2 -> [qdot_sgn2]
  [qdot_sgn1] -> Terminator1/1
  tau_measured/1 -> [tau_measured]
  [psi2] -> tau seg2 bias LUT/2(psi seg2)
  [qdot_sgn2] -> tau seg2 bias LUT/1(q dot seg2)
  Constant/1 -> Mux/1
  tau seg2 bias LUT/1(tau bias seg2) -> Mux/2
  Mux/1 -> Sum/2  "tau bias"
  [tau_measured] -> Sum/1
  Sum/1 -> tau_comp/1
